simulink model "quad_copter"  (R2016a)
settings: Solver=VariableStepAuto  StartTime=0.0  StopTime=70  RelTol=1e-3
undefined symbols (not defined in the file): DiscIntNeverNeededParam, HybridVRFTController, InnerReferenceModel, InnerReferenceModel_dt, Mixer, OptimalInnerController, OptimalOuterController, OuterReferenceModel, PitchRateModel_dt, PitchRateModel_tf, Ri_dt, Ri_tf, Ro_tf, step_size, time_step, Ts
settings Model: Creator=tibo  LastModifiedBy=tibo

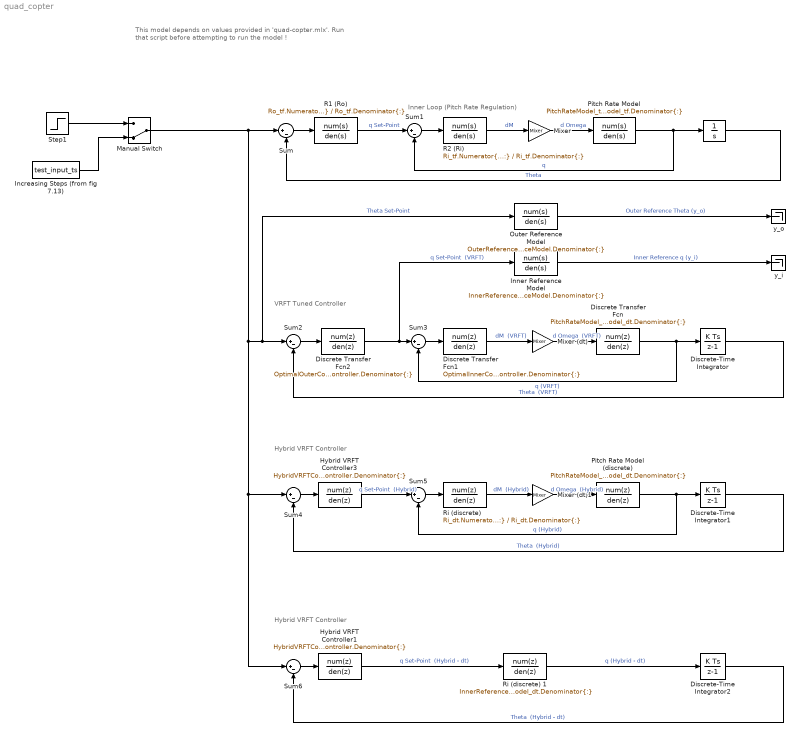
== system quad_copter ==
  note: VRFT Tuned Controller
  note: This model depends on values provided in 'quad-copter.mlx'.
      | Run that script before attempting to run the model !
  note: Inner Loop (Pitch Rate Regulation)
  note: Hybrid VRFT Controller
  note: Hybrid VRFT Controller
  " " : Integrator  ContinuousStateAttributes='PitchAngle'
  Discrete Transfer Fcn : DiscreteTransferFcn  Numerator=PitchRateModel_dt.Numerator{:}  Denominator=PitchRateModel_dt.Denominator{:}  SampleTime=Ts
  Discrete Transfer Fcn1 : DiscreteTransferFcn  Numerator=OptimalInnerController.Numerator{:}  Denominator=OptimalInnerController.Denominator{:}  SampleTime=Ts
  Discrete Transfer Fcn2 : DiscreteTransferFcn  Numerator=OptimalOuterController.Numerator{:}  Denominator=OptimalOuterController.Denominator{:}  SampleTime=Ts
  Discrete-Time Integrator : DiscreteIntegrator  InitialConditionSetting=State (most efficient)  SampleTime=Ts  ICPrevOutput=DiscIntNeverNeededParam  ICPrevScaledInput=DiscIntNeverNeededParam
  Discrete-Time Integrator1 : DiscreteIntegrator  InitialConditionSetting=State (most efficient)  SampleTime=Ts  ICPrevOutput=DiscIntNeverNeededParam  ICPrevScaledInput=DiscIntNeverNeededParam
  Discrete-Time Integrator2 : DiscreteIntegrator  InitialConditionSetting=State (most efficient)  SampleTime=Ts  ICPrevOutput=DiscIntNeverNeededParam  ICPrevScaledInput=DiscIntNeverNeededParam
  Hybrid VRFT Controller1 : DiscreteTransferFcn  Numerator=HybridVRFTController.Numerator{:}  Denominator=HybridVRFTController.Denominator{:}  SampleTime=Ts
  Hybrid VRFT Controller3 : DiscreteTransferFcn  Numerator=HybridVRFTController.Numerator{:}  Denominator=HybridVRFTController.Denominator{:}  SampleTime=Ts
  Increasing Steps (from fig 7.13) : FromWorkspace  VariableName=test_input_ts  SampleTime=time_step  OutputAfterFinalValue=Holding final value
  Inner Reference Model : TransferFcn  Numerator=InnerReferenceModel.Numerator{:}  Denominator=InnerReferenceModel.Denominator{:}
  Manual Switch : ManualSwitch  CurrentSetting=0
  "Mixer " : Gain  Gain=Mixer
  Mixer (dt) : Gain  Gain=Mixer
  Mixer (dt)1 : Gain  Gain=Mixer
  Outer Reference Model : TransferFcn  Numerator=OuterReferenceModel.Numerator{:}  Denominator=OuterReferenceModel.Denominator{:}
  "Pitch Rate Model " : TransferFcn  Numerator=PitchRateModel_tf.Numerator{:}  Denominator=PitchRateModel_tf.Denominator{:}  ContinuousStateAttributes='PitchRate'
  "Pitch Rate Model (discrete) " : DiscreteTransferFcn  Numerator=PitchRateModel_dt.Numerator{:}  Denominator=PitchRateModel_dt.Denominator{:}  SampleTime=Ts
  "R1 (Ro) " : TransferFcn  Numerator=Ro_tf.Numerator{:}  Denominator=Ro_tf.Denominator{:}
  "R2 (Ri) " : TransferFcn  Numerator=Ri_tf.Numerator{:}  Denominator=Ri_tf.Denominator{:}
  "Ri (discrete) " : DiscreteTransferFcn  Numerator=Ri_dt.Numerator{:}  Denominator=Ri_dt.Denominator{:}  SampleTime=Ts
  Ri (discrete) 1 : DiscreteTransferFcn  Numerator=InnerReferenceModel_dt.Numerator{:}  Denominator=InnerReferenceModel_dt.Denominator{:}  SampleTime=Ts
  Step1 : Step  After=step_size  SampleTime=0
  Sum{,1..6} (7 alike) : Sum  Inputs=|+-
  y_i : Terminator
  y_o : Terminator
  wires:
  Sum/1 -> "R1 (Ro) "/1
  "R1 (Ro) "/1 -> Sum1/1  "q Set-Point"
  "R2 (Ri) "/1 -> "Mixer "/1  "dM"
  "Mixer "/1 -> "Pitch Rate Model "/1  "d Omega"
  "Pitch Rate Model "/1 -> Sum1/2, " "/1  "q"
  " "/1 -> Sum/2  "Theta"
  Increasing Steps (from fig 7.13)/1 -> Manual Switch/2
  Step1/1 -> Manual Switch/1
  Sum1/1 -> "R2 (Ri) "/1
  Sum2/1 -> Discrete Transfer Fcn2/1
  Discrete Transfer Fcn2/1 -> Inner Reference Model/1, Sum3/1  "q Set-Point  (VRFT)"
  Discrete Transfer Fcn1/1 -> Mixer (dt)/1  "dM  (VRFT)"
  Mixer (dt)/1 -> Discrete Transfer Fcn/1  "d Omega  (VRFT)"
  Discrete Transfer Fcn/1 -> Discrete-Time Integrator/1, Sum3/2  "q (VRFT)"
  Discrete-Time Integrator/1 -> Sum2/2  "Theta  (VRFT)"
  Sum3/1 -> Discrete Transfer Fcn1/1
  Outer Reference Model/1 -> y_o/1  "Outer Reference Theta (y_o)"
  Inner Reference Model/1 -> y_i/1  "Inner Reference q (y_i)"
  Sum4/1 -> Hybrid VRFT Controller3/1
  Hybrid VRFT Controller3/1 -> Sum5/1  "q Set-Point  (Hybrid)"
  "Ri (discrete) "/1 -> Mixer (dt)1/1  "dM  (Hybrid)"
  Mixer (dt)1/1 -> "Pitch Rate Model (discrete) "/1  "d Omega  (Hybrid)"
  "Pitch Rate Model (discrete) "/1 -> Discrete-Time Integrator1/1, Sum5/2  "q (Hybrid)"
  Discrete-Time Integrator1/1 -> Sum4/2  "Theta  (Hybrid)"
  Sum5/1 -> "Ri (discrete) "/1
  Manual Switch/1 -> Sum4/1, Sum6/1, Outer Reference Model/1, Sum2/1, Sum/1  "Theta Set-Point"
  Sum6/1 -> Hybrid VRFT Controller1/1
  Discrete-Time Integrator2/1 -> Sum6/2  "Theta  (Hybrid - dt)"
  Hybrid VRFT Controller1/1 -> Ri (discrete) 1/1  "q Set-Point  (Hybrid - dt)"
  Ri (discrete) 1/1 -> Discrete-Time Integrator2/1  "q (Hybrid - dt)"
